simulink model "SD2231_Lab1m"  (R2018b)
settings: Solver=ode45  StartTime=0.0  StopTime=inf  RelTol=1e-3  EnableMultiTasking=on
values from neighbouring files (symbols this model uses):
  K_brake = K_brake(3)    [initial.m]    (also in initialm.m)
  K_em = K_em(3)    [initial.m]    (also in initialm.m)
  Kd_brake = 0    [initial.m]    (also in initialm.m)
  Kd_brake_r = 0.01    [initialm.m]
  Kd_em = 0.0    (= 0)    [initial.m]    (also in initialm.m)
  Ki_brake = 0    [initial.m]    (also in initialm.m = 22.5)
  Ki_brake_r = 13.5    [initialm.m]
  Ki_em = 1.2    [initial.m]    (also in initialm.m = 12.5)
  Kp_brake = 0    [initial.m]    (also in initialm.m = 5.5)
  Kp_brake_r = 4.25    [initialm.m]
  Kp_em = 6.5    [initial.m]    (also in initialm.m = 2.5)
undefined symbols (not defined in the file or in its folder): ABS_slip_refF, ABS_slip_refR, DiscIntNeverNeededParam, TCS_slip_ref, Veh
libraries: CarMaker4SL x37, simulink x9, autolibmappedmotor x2
(part 1 of 2)
settings Model: ExtModeAutoUpdateStatusClock=off  Creator=fh  LastModifiedBy=anirv
settings DataIOCC: LimitDataPoints=on  SaveFormat=Array  SignalLoggingName=sigsOut
settings OptimizationCC: BooleanDataType=off  ExpressionDepthLimit=2147483647  InitFltsAndDblsToZero=on  LifeSpan=inf
settings DebuggingCC: SaveWithParameterizedLinksMsg=none  UnderspecifiedInitializationDetection=Classic  MergeDetectMultiDrivingBlocksExec=none  SignalResolutionControl=TryResolveAllWithWarning  MultiTaskDSMMsg=warning  MultiTaskCondExecSysMsg=none  FcnCallInpInsideContextMsg=warning  StateNameClashWarn=warning  SFUnexpectedBacktrackingDiag=warning  SFNoUnconditionalDefaultTransitionDiag=warning
settings HardwareCC: ProdBitPerPointer=32  ProdBitPerSizeT=32  ProdBitPerPtrDiffT=32  ProdLargestAtomicFloat=None  ProdIntDivRoundTo=Undefined  ProdEndianess=Unspecified  ProdWordSize=32  ProdHWDeviceType=32-bit Generic  TargetUnknown=on
settings ModelReferenceCC: PropagateSignalLabelsOutOfModel=off
settings SFSimCC: SimUseLocalCustomCode=off
settings RTWCC: RTWUseLocalCustomCode=off
settings CodeAppCC: MaxIdLength=63  StateflowObjectComments=on
settings GRTTargetCC: TargetFcnLib=ansi_tfl_tmw.mat  TargetLangStandard=C89/C90 (ANSI)  GeneratePreprocessorConditionals=Disable all  CombineOutputUpdateFcns=off  GRTInterface=on
settings ConfigComp: CovMetricSettings=dw  CovHtmlReporting=on  CovSaveCumulativeToWorkspaceVar=on  CovSaveSingleToWorkspaceVar=on  CovExternalEMLEnable=off

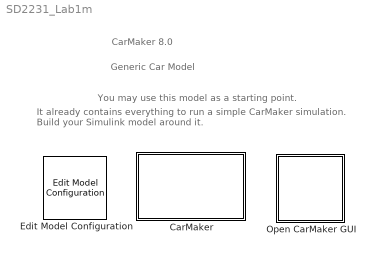
== system SD2231_Lab1m ==
  note: Generic Car Model
  note: You may use this model as a starting point.
  note: It already contains everything to run a simple CarMaker simulation.
      | Build your Simulink model around it.
  note: CarMaker 8.0
  CarMaker : Subsystem  TreatAsAtomicUnit=on
      mask Display: image(imread('CarMakerSys.png'));
  Edit Model Configuration : CarMaker4SL/Edit Model Configuration  SFunctionModules=''
  Open CarMaker GUI : Subsystem  LoadFcn=if ~length(which('cmself')), cmenv; end
      settings: OpenFcn=cmblockmagic('gui_fix_display'); CM_Simulink
      mask Display: image(imread('CarMakerGUI.png'));

== system SD2231_Lab1m/CarMaker ==
  Bus Creator : BusCreator  Inputs=6
  CM_FIRST : Subsystem
  CM_LAST : Subsystem
  CarMaker data : Subsystem
  DrivMan : Subsystem
  Ground : Ground
  IPG Vehicle : Subsystem  TreatAsAtomicUnit=on
  Road friction : Subsystem
  Terminator : Terminator
  Used friction mapping : Subsystem
  VehicleControl : Subsystem
  Your ABS Controller : Subsystem
  Your Traction Controller : Subsystem
  Your observer : Subsystem
  wires:
  DrivMan/2(DrivMan.Out) -> VehicleControl/2(DrivMan.In)
  DrivMan/1(Sync_Out) -> VehicleControl/1(Sync_In)
  CM_FIRST/2(Env.Misc) -> DrivMan/2(Env.Misc)
  CM_FIRST/1(Sync_Out) -> DrivMan/1(Sync_In)
  CM_LAST/1(Sync_Out) -> Terminator/1
  Ground/1 -> CM_FIRST/1(Sync_In)
  IPG Vehicle/1(Sync_Out) -> CM_LAST/1(Sync_In)
  VehicleControl/1(Sync_Out) -> IPG Vehicle/1(Sync_In)
  VehicleControl/3(VhclCtrl.Steering) -> IPG Vehicle/3(VhclCtrl.Steering)
  VehicleControl/4(Vhcl.Wheel.In) -> IPG Vehicle/4(Vhcl.Wheel.In)
  VehicleControl/5(Vhcl.Misc) -> IPG Vehicle/5(Vhcl.Misc)
  VehicleControl/6(VhclCtrl.Brake) -> IPG Vehicle/6(VhclCtrl.Brake)
  VehicleControl/7(VhclCtrl.PT) -> IPG Vehicle/7(VhclCtrl.PT)
  VehicleControl/2(Vhcl.Model.Source) -> IPG Vehicle/2(Vhcl.Model.Source)
  Your ABS Controller/1(FLBrakeAdjust (0-1)) -> Bus Creator/3
  Your ABS Controller/2(FRBrakeAdjust (0-1)) -> Bus Creator/4
  Your ABS Controller/3(RLBrakeAdjust (0-1)) -> Bus Creator/5
  Your ABS Controller/4(RRBrakeAdjust (0-1)) -> Bus Creator/6
  Bus Creator/1 -> IPG Vehicle/8(SD2231.data)
  CarMaker data/1(CarMaker bus data) -> Your observer/1(CarMaker bus data)
  Your observer/1(CarMaker bus data out) -> Your ABS Controller/1(CarMaker Bus data), Your Traction Controller/1(CarMaker Bus data)
  Your observer/2(Tyre slip bus data out) -> Your ABS Controller/2(TyreSlipBusDataOut), Your Traction Controller/2("TyreSlipBusDataOut "), Used friction mapping/1(Tyre slip bus data out)
  Your Traction Controller/1(LR TrqReqSignal (0-1)) -> Bus Creator/1
  Your Traction Controller/2(RR TrqReqSignal (0-1)) -> Bus Creator/2

== system SD2231_Lab1m/Open CarMaker GUI ==
  S-Function : S-Function  FunctionName=cm_gui  SFunctionDeploymentMode=off  EnableBusSupport=off

== system SD2231_Lab1m/CarMaker/CM_FIRST ==
  Sync_In : Inport
  BusCreator1 : BusCreator  Inputs=8
  BusCreator2 : BusCreator  Inputs=6
  Demux1 : Demux  Outputs=14
  Environment : S-Function  FunctionName=CM_Sfun  Parameters='Environment'  SFunctionDeploymentMode=off  EnableBusSupport=off
  IoIn : S-Function  FunctionName=CM_Sfun  Parameters='IoIn'  SFunctionDeploymentMode=off  EnableBusSupport=off
  Terminator : Terminator
  Sync_Out : Outport
  Env.Misc : Outport  Port=2
  wires:
  BusCreator2/1 -> Terminator/1  "IF Environment (in)"
  BusCreator1/1 -> Env.Misc/1
  Demux1/14 -> BusCreator2/6  "Env sRoad"
  Demux1/13 -> BusCreator2/5  "Env PoI_GCS Elev"
  Demux1/12 -> BusCreator2/4  "Env PoI_GCS Lat"
  Demux1/11 -> BusCreator2/3  "Env PoI_GCS Long"
  Demux1/10 -> BusCreator2/2  "Env Time"
  Demux1/9 -> BusCreator2/1  "Env yDay"
  Demux1/8 -> BusCreator1/8  "Env WindVel_tot z"
  Demux1/7 -> BusCreator1/7  "Env WindVel_tot y"
  Demux1/6 -> BusCreator1/6  "Env WindVel_tot x"
  Demux1/5 -> BusCreator1/5  "Env SolarRadiation"
  Demux1/4 -> BusCreator1/4  "Env AirHumidity"
  Demux1/3 -> BusCreator1/3  "Env AirPressure"
  Demux1/2 -> BusCreator1/2  "Env AirDensity"
  Demux1/1 -> BusCreator1/1  "Env Temperature"
  Environment/2 -> Demux1/1
  Environment/1 -> Sync_Out/1
  IoIn/1 -> Environment/1
  Sync_In/1 -> IoIn/1

== system SD2231_Lab1m/CarMaker/CM_LAST ==
  Sync_In : Inport
  CM_User : S-Function  FunctionName=CM_Sfun  Parameters='CM_User'  SFunctionDeploymentMode=off  EnableBusSupport=off
  IoOut : S-Function  FunctionName=CM_Sfun  Parameters='IoOut'  SFunctionDeploymentMode=off  EnableBusSupport=off
  Sync_Out : Outport
  wires:
  IoOut/1 -> Sync_Out/1
  CM_User/1 -> IoOut/1
  Sync_In/1 -> CM_User/1

== system SD2231_Lab1m/CarMaker/CarMaker data ==
  Brake pedal [0-1] : CarMaker4SL/Read CM Dict  xname=Driver.Brake  xsync=off
  Bus Creator : BusCreator  Inputs=15
  Distance [m] : CarMaker4SL/Read CM Dict  xname=Vhcl.Distance  xsync=off
  FL Tyre radius [m] : CarMaker4SL/Read CM Dict  xname=Car.WFL.Radius  xsync=off
  FL Tyre rot. vel. [rad/s] : CarMaker4SL/Read CM Dict  xname=Car.WheelSpd_FL  xsync=off
  FR Tyre radius [m] : CarMaker4SL/Read CM Dict  xname=Car.WFR.Radius  xsync=off
  FR Tyre rot. vel. [rad/s] : CarMaker4SL/Read CM Dict  xname=Car.WheelSpd_FR  xsync=off
  RL Tyre radius [m] : CarMaker4SL/Read CM Dict  xname=Car.WRL.Radius  xsync=off
  RL Tyre rot. vel. [rad/s] : CarMaker4SL/Read CM Dict  xname=Car.WheelSpd_RL  xsync=off
  RR Tyre radius [m] : CarMaker4SL/Read CM Dict  xname=Car.WRR.Radius  xsync=off
  RR Tyre rot. vel. [rad/s] : CarMaker4SL/Read CM Dict  xname=Car.WheelSpd_RR  xsync=off
  Steering wheel angle [rad] : CarMaker4SL/Read CM Dict  xname=Driver.Steer.Ang  xsync=off
  Throttle [0-1] : CarMaker4SL/Read CM Dict  xname=Driver.Gas  xsync=off
  Vehicle Yaw Rate [rad/s] : CarMaker4SL/Read CM Dict  xname=Car.YawRate  xsync=off
  Vehicle ax [m/s^2] : CarMaker4SL/Read CM Dict  xname=Car.ax  xsync=off
  Vehicle velocity [m/s] : CarMaker4SL/Read CM Dict  xname=Car.v  xsync=off
  CarMaker bus data : Outport
  wires:
  RR Tyre rot. vel. [rad/s]/1 -> Bus Creator/8  "RR Tyre rot vel"
  RL Tyre rot. vel. [rad/s]/1 -> Bus Creator/7  "RL Tyre rot vel"
  Distance [m]/1 -> Bus Creator/4  "Distance"
  FR Tyre rot. vel. [rad/s]/1 -> Bus Creator/6  "FR Tyre rot vel"
  Brake pedal [0-1]/1 -> Bus Creator/2  "Brake pedal"
  Vehicle ax [m/s^2]/1 -> Bus Creator/9  "Vehicle ax"
  Steering wheel angle [rad]/1 -> Bus Creator/3  "Steering wheel angle"
  Throttle [0-1]/1 -> Bus Creator/1  "Throttle"
  Vehicle velocity [m/s]/1 -> Bus Creator/10  "Vehicle velocity"
  FL Tyre rot. vel. [rad/s]/1 -> Bus Creator/5  "FL Tyre rot vel"
  Vehicle Yaw Rate [rad/s]/1 -> Bus Creator/11  "Vehicle Yaw Rate"
  FL Tyre radius [m]/1 -> Bus Creator/12  "FL Tyre radius"
  FR Tyre radius [m]/1 -> Bus Creator/13  "FR Tyre radius"
  RL Tyre radius [m]/1 -> Bus Creator/14  "RL Tyre radius"
  RR Tyre radius [m]/1 -> Bus Creator/15  "RR Tyre radius"
  Bus Creator/1 -> CarMaker bus data/1  "CarMaker bus data"

== system SD2231_Lab1m/CarMaker/DrivMan ==
  note: There's rarely a reason to override DrivMan signals.
      | Use the VehicleControl interface for this purpose.
  Sync_In : Inport
  Env.Misc : Inport  Port=2
  BusCreator : BusCreator  Inputs=17
  Demux : Demux  Outputs=17
  DrivMan : S-Function  FunctionName=CM_Sfun  Parameters='DrivMan'  SFunctionDeploymentMode=off  EnableBusSupport=off
  Sync_Out : Outport
  DrivMan.Out : Outport  Port=2
  wires:
  Demux/17 -> BusCreator/17  "DrivMan Steering Trq"
  Demux/16 -> BusCreator/16  "DrivMan Steering AngAcc"
  Demux/15 -> BusCreator/15  "DrivMan Steering AngVel"
  Demux/14 -> BusCreator/14  "DrivMan Steering Ang"
  Demux/13 -> BusCreator/13  "DrivMan Gas"
  Demux/12 -> BusCreator/12  "DrivMan Clutch"
  Demux/11 -> BusCreator/11  "DrivMan BrakePark"
  Demux/10 -> BusCreator/10  "DrivMan Brake"
  Demux/9 -> BusCreator/9  "DrivMan GearNo"
  Demux/8 -> BusCreator/8  "DrivMan SelectorCtrl"
  Demux/7 -> BusCreator/7  "DrivMan UserSignal4"
  Demux/6 -> BusCreator/6  "DrivMan UserSignal3"
  Demux/5 -> BusCreator/5  "DrivMan UserSignal2"
  Demux/4 -> BusCreator/4  "DrivMan UserSignal1"
  Demux/3 -> BusCreator/3  "DrivMan UserSignal0"
  Demux/2 -> BusCreator/2  "DrivMan Key"
  Demux/1 -> BusCreator/1  "DrivMan SST"
  Env.Misc/1 -> DrivMan/2
  Sync_In/1 -> DrivMan/1
  DrivMan/1 -> Sync_Out/1
  BusCreator/1 -> DrivMan.Out/1
  DrivMan/2 -> Demux/1

== system SD2231_Lab1m/CarMaker/IPG Vehicle ==
  Sync_In : Inport
  Vhcl.Model.Source : Inport  Port=2
  VhclCtrl.Steering : Inport  Port=3
  Vhcl.Wheel.In : Inport  Port=4
  Vhcl.Misc : Inport  Port=5
  VhclCtrl.Brake : Inport  Port=6
  VhclCtrl.PT : Inport  Port=7
  SD2231.data : Inport  Port=8
  Brake1 : Subsystem
  CarAndTrailer1 : Subsystem
  PowerTrain1 : Subsystem
  Stop Simulation : Stop
  VehicleSource_BuiltIn : simulink/Logic and Bit Operations/Compare To Constant  relop=~=  const=1  OutDataTypeStr=boolean  ZeroCross=off
  Sync_Out : Outport
  wires:
  CarAndTrailer1/1(Sync_Out) -> Brake1/1(Sync_In)
  CarAndTrailer1/2(Brake.IF.In) -> Brake1/2(Brake.IF.In)
  VhclCtrl.Brake/1 -> Brake1/3(VhclCtrl.Brake)
  PowerTrain1/1(Sync_Out) -> Sync_Out/1
  Vhcl.Misc/1 -> CarAndTrailer1/4(Vhcl.Misc)
  Vhcl.Wheel.In/1 -> CarAndTrailer1/3(Vhcl.Wheel.In)
  VhclCtrl.Steering/1 -> CarAndTrailer1/2(VhclCtrl.Steering)
  Sync_In/1 -> CarAndTrailer1/1(Sync_In)
  Vhcl.Model.Source/1 -> VehicleSource_BuiltIn/1
  VehicleSource_BuiltIn/1 -> Stop Simulation/1
  Brake1/1(Sync_Out) -> PowerTrain1/1(Sync_In)
  Brake1/2(Vhcl.Wheel.PT) -> PowerTrain1/2(Vhcl.Wheel.PT)
  VhclCtrl.PT/1 -> PowerTrain1/3(VhclCtrl.PT)
  Brake1/3(Brake.IF.Out) -> PowerTrain1/4(Brake.IF.Out)
  CarAndTrailer1/3(Car.Trq_T2W) -> PowerTrain1/5(Car.TrqT2W)
  SD2231.data/1 -> Brake1/4(SD2231.Data), PowerTrain1/6(SD2232.data)

== system SD2231_Lab1m/CarMaker/Road friction ==
  Constant : Constant  Value=Veh.mu
  Write CM Dict : CarMaker4SL/Write CM Dict  xname=Car.muRoadFL  xsync=off
  Write CM Dict1 : CarMaker4SL/Write CM Dict  xname=Car.muRoadFR  xsync=off
  Write CM Dict2 : CarMaker4SL/Write CM Dict  xname=Car.muRoadRL  xsync=off
  Write CM Dict3 : CarMaker4SL/Write CM Dict  xname=Car.muRoadRR  xsync=off
  wires:
  Constant/1 -> Write CM Dict3/1, Write CM Dict2/1, Write CM Dict1/1, Write CM Dict/1

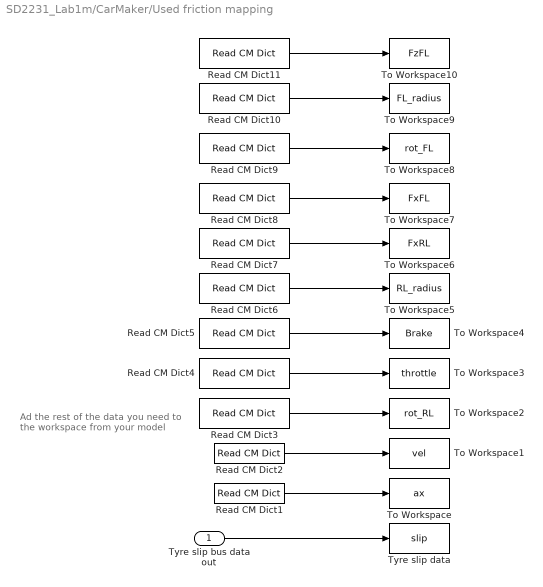
== system SD2231_Lab1m/CarMaker/Used friction mapping ==
  note: Ad the rest of the data you need to
      | the workspace from your model
  Tyre slip bus data out : Inport
  Read CM Dict1 : CarMaker4SL/Read CM Dict  xname=Car.ax  xsync=off
  Read CM Dict10 : CarMaker4SL/Read CM Dict  xname=Car.WRL.Radius  xsync=off
  Read CM Dict11 : CarMaker4SL/Read CM Dict  xname=Car.FzFL  xsync=off
  Read CM Dict2 : CarMaker4SL/Read CM Dict  xname=Car.v  xsync=off
  Read CM Dict3 : CarMaker4SL/Read CM Dict  xname=Car.WheelSpd_RL  xsync=off
  Read CM Dict4 : CarMaker4SL/Read CM Dict  xname=Driver.Gas  xsync=off
  Read CM Dict5 : CarMaker4SL/Read CM Dict  xname=Driver.Brake  xsync=off
  Read CM Dict6 : CarMaker4SL/Read CM Dict  xname=Car.WRL.Radius  xsync=off
  Read CM Dict7 : CarMaker4SL/Read CM Dict  xname=Car.FxRL  xsync=off
  Read CM Dict8 : CarMaker4SL/Read CM Dict  xname=Car.FxFL  xsync=off
  Read CM Dict9 : CarMaker4SL/Read CM Dict  xname=Car.WheelSpd_FL  xsync=off
  To Workspace : ToWorkspace  VariableName=ax  SampleTime=-1
  To Workspace1 : ToWorkspace  VariableName=vel  SampleTime=-1
  To Workspace10 : ToWorkspace  VariableName=FzFL  SampleTime=-1
  To Workspace2 : ToWorkspace  VariableName=rot_RL  SampleTime=-1
  To Workspace3 : ToWorkspace  VariableName=throttle  SampleTime=-1
  To Workspace4 : ToWorkspace  VariableName=Brake  SampleTime=-1
  To Workspace5 : ToWorkspace  VariableName=RL_radius  SampleTime=-1
  To Workspace6 : ToWorkspace  VariableName=FxRL  SampleTime=-1
  To Workspace7 : ToWorkspace  VariableName=FxFL  SampleTime=-1
  To Workspace8 : ToWorkspace  VariableName=rot_FL  SampleTime=-1
  To Workspace9 : ToWorkspace  VariableName=FL_radius  SampleTime=-1
  Tyre slip data : ToWorkspace  VariableName=slip  SampleTime=-1
  wires:
  Read CM Dict1/1 -> To Workspace/1
  Tyre slip bus data out/1 -> Tyre slip data/1
  Read CM Dict2/1 -> To Workspace1/1
  Read CM Dict3/1 -> To Workspace2/1
  Read CM Dict4/1 -> To Workspace3/1
  Read CM Dict5/1 -> To Workspace4/1
  Read CM Dict6/1 -> To Workspace5/1
  Read CM Dict8/1 -> To Workspace7/1
  Read CM Dict7/1 -> To Workspace6/1
  Read CM Dict9/1 -> To Workspace8/1
  Read CM Dict10/1 -> To Workspace9/1
  Read CM Dict11/1 -> To Workspace10/1

== system SD2231_Lab1m/CarMaker/VehicleControl ==
  note: <Your model here>
  note: When implementing a vehicle control model,
      | be sure to add '-disablevehiclecontrol' to the command line arguments
      | in the CarMaker Model Configuration block.
      | Otherwise your model will possibly not see the original DrivMan signals
      | on its inputs, but those of a currently activated C-coded vehicle control model instead.
  Sync_In : Inport
  DrivMan.In : Inport  Port=2
  Bus Creator2 : BusCreator  Inputs=2
  CreateBus Vhcl.Misc : Subsystem
  CreateBus Vhcl.Wheel.In : Subsystem
  CreateBus VhclCtrl : Subsystem
  CreateBus VhclCtrl.PT : Subsystem
  CreateBus VhclCtrl.Steering : Subsystem
  Demux2 : Demux  Outputs=2
  VehicleControl : S-Function  FunctionName=CM_Sfun  Parameters='VehicleControl'  SFunctionDeploymentMode=off  EnableBusSupport=off
  VehicleControlUpd : S-Function  FunctionName=CM_Sfun  Parameters='VehicleControlUpd'  SFunctionDeploymentMode=off  EnableBusSupport=off
  Sync_Out : Outport
  Vhcl.Model.Source : Outport  Port=2
  VhclCtrl.Steering : Outport  Port=3
  Vhcl.Wheel.In : Outport  Port=4
  Vhcl.Misc : Outport  Port=5
  VhclCtrl.Brake : Outport  Port=6
  VhclCtrl.PT : Outport  Port=7
  wires:
  CreateBus VhclCtrl/1(Out) -> VehicleControlUpd/2
  VehicleControl/2 -> CreateBus VhclCtrl/1(In)
  VehicleControlUpd/2 -> Vhcl.Model.Source/1
  VehicleControlUpd/4 -> CreateBus Vhcl.Wheel.In/1(In1)
  VehicleControlUpd/5 -> CreateBus Vhcl.Misc/1(In1)
  VehicleControlUpd/6 -> Demux2/1
  VehicleControlUpd/7 -> CreateBus VhclCtrl.PT/1(In1)
  VehicleControlUpd/3 -> CreateBus VhclCtrl.Steering/1(In1)
  CreateBus Vhcl.Misc/1(Out1) -> Vhcl.Misc/1
  CreateBus Vhcl.Wheel.In/1(Out1) -> Vhcl.Wheel.In/1
  DrivMan.In/1 -> VehicleControl/2
  VehicleControl/1 -> VehicleControlUpd/1
  Sync_In/1 -> VehicleControl/1
  CreateBus VhclCtrl.PT/1(Out1) -> VhclCtrl.PT/1
  Bus Creator2/1 -> VhclCtrl.Brake/1
  CreateBus VhclCtrl.Steering/1(Out1) -> VhclCtrl.Steering/1
  VehicleControlUpd/1 -> Sync_Out/1
  Demux2/2 -> Bus Creator2/2  "VhclCtrl BrakePark"
  Demux2/1 -> Bus Creator2/1  "VhclCtrl Brake"

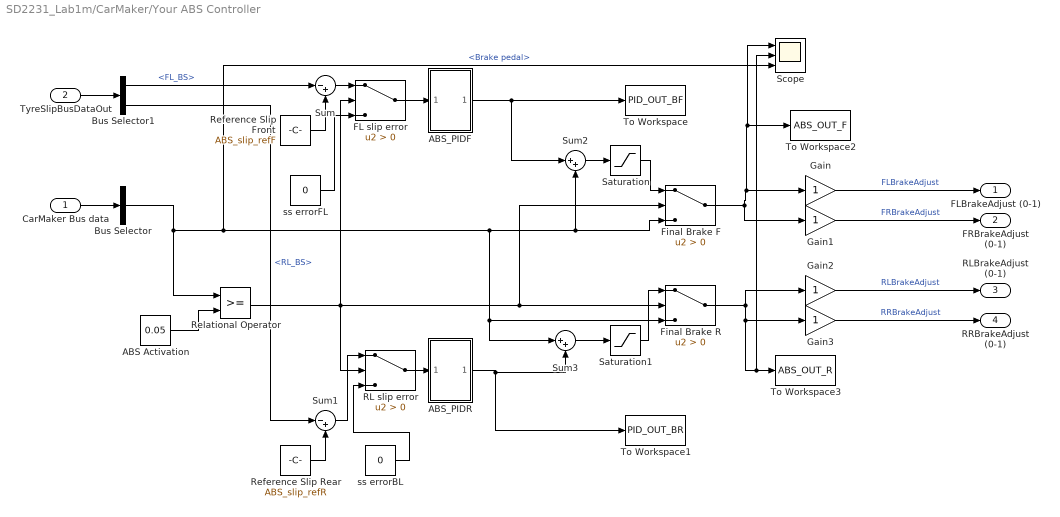
== system SD2231_Lab1m/CarMaker/Your ABS Controller ==
  CarMaker Bus data : Inport
  TyreSlipBusDataOut : Inport  Port=2
  ABS Activation : Constant  Value=0.05
  ABS_PIDF : Subsystem
  ABS_PIDR : Subsystem
  Bus Selector : BusSelector  OutputSignals=Brake pedal
  Bus Selector1 : BusSelector  OutputSignals=FL_BS,RL_BS
  FL slip error : Switch  Criteria=u2 > Threshold
  Final Brake F : Switch  Criteria=u2 > Threshold
  Final Brake R : Switch  Criteria=u2 > Threshold
  Gain{,1..3} (4 alike) : Gain
  RL slip error : Switch  Criteria=u2 > Threshold
  Reference Slip Rear : Constant  Value=ABS_slip_refR
  Reference Slip Front : Constant  Value=ABS_slip_refF
  Relational Operator : RelationalOperator  OutDataTypeStr=boolean  RndMeth=Simplest
  Saturation : Saturate  UpperLimit=1  LowerLimit=0  LinearizeAsGain=off  ZeroCross=off
  Saturation1 : Saturate  UpperLimit=1  LowerLimit=0  LinearizeAsGain=off  ZeroCross=off
  Scope : Scope  NumInputPorts=3
  Sum : Sum  Inputs=|-+
  Sum1 : Sum  Inputs=|-+
  Sum2 : Sum  Inputs=|++
  Sum3 : Sum  Inputs=|++
  To Workspace : ToWorkspace  VariableName=PID_OUT_BF  SaveFormat=Timeseries  SampleTime=-1
  To Workspace1 : ToWorkspace  VariableName=PID_OUT_BR  SaveFormat=Timeseries  SampleTime=-1
  To Workspace2 : ToWorkspace  VariableName=ABS_OUT_F  SaveFormat=Timeseries  SampleTime=-1
  To Workspace3 : ToWorkspace  VariableName=ABS_OUT_R  SaveFormat=Timeseries  SampleTime=-1
  ss errorBL : Constant  Value=0
  ss errorFL : Constant  Value=0
  FLBrakeAdjust (0-1) : Outport
  FRBrakeAdjust (0-1) : Outport  Port=2
  RLBrakeAdjust (0-1) : Outport  Port=3
  RRBrakeAdjust (0-1) : Outport  Port=4
  wires:
  CarMaker Bus data/1 -> Bus Selector/1
  Gain/1 -> FLBrakeAdjust (0-1)/1  "FLBrakeAdjust"
  Gain1/1 -> FRBrakeAdjust (0-1)/1  "FRBrakeAdjust"
  Gain2/1 -> RLBrakeAdjust (0-1)/1  "RLBrakeAdjust"
  Gain3/1 -> RRBrakeAdjust (0-1)/1  "RRBrakeAdjust"
  ABS Activation/1 -> Relational Operator/2
  TyreSlipBusDataOut/1 -> Bus Selector1/1
  Reference Slip Front/1 -> Sum/2
  Reference Slip Rear/1 -> Sum1/2
  Relational Operator/1 -> RL slip error/2, Final Brake R/2, Final Brake F/2, FL slip error/2
  ABS_PIDR/1(Out1) -> Sum3/2, To Workspace1/1
  Bus Selector1/1 -> Sum/1  "<FL_BS>"
  Bus Selector/1 -> Relational Operator/1, Scope/3, Sum3/1, Final Brake R/3, Sum2/2, Final Brake F/3  "<Brake pedal>"
  Bus Selector1/2 -> Sum1/1  "<RL_BS>"
  Final Brake F/1 -> Scope/1, To Workspace2/1, Gain/1, Gain1/1
  Final Brake R/1 -> Scope/2, To Workspace3/1, Gain3/1, Gain2/1
  Sum2/1 -> Saturation/1
  Saturation/1 -> Final Brake F/1
  Sum3/1 -> Saturation1/1
  Saturation1/1 -> Final Brake R/1
  ss errorFL/1 -> FL slip error/3
  Sum/1 -> FL slip error/1
  FL slip error/1 -> ABS_PIDF/1(In1)
  Sum1/1 -> RL slip error/1
  RL slip error/1 -> ABS_PIDR/1(In1)
  ss errorBL/1 -> RL slip error/3
  ABS_PIDF/1(Out1) -> Sum2/1, To Workspace/1

== system SD2231_Lab1m/CarMaker/Your Traction Controller ==
  CarMaker Bus data : Inport
  "TyreSlipBusDataOut " : Inport  Port=2
  Bus Selector : BusSelector  OutputSignals=Throttle
  Bus Selector1 : BusSelector  OutputSignals=RL_TS
  Constant : Constant  Value=0
  Gain : Gain
  Gain1 : Gain
  Relational Operator : RelationalOperator  Operator=<=  OutDataTypeStr=boolean  RndMeth=Simplest
  SS error : Constant  Value=0
  Saturation : Saturate  UpperLimit=1  LowerLimit=0  LinearizeAsGain=off  ZeroCross=off
  "Slip Check " : Switch  Criteria=u2 > Threshold  Threshold=0.01
  Slip reference : Constant  Value=TCS_slip_ref
  Sum : Sum  Inputs=|-+
  Sum1 : Sum  Inputs=|++
  TCS Active : Switch  Criteria=u2 > Threshold  Threshold=0.4
  TCS_PID : Subsystem
  Throttle Check : Switch  Criteria=u2 > Threshold
  To Workspace : ToWorkspace  VariableName=PID_out  SaveFormat=Timeseries  SampleTime=-1
  To Workspace1 : ToWorkspace  VariableName=TCS_out  SaveFormat=Timeseries  SampleTime=-1
  LR TrqReqSignal (0-1) : Outport
  RR TrqReqSignal (0-1) : Outport  Port=2
  wires:
  CarMaker Bus data/1 -> Bus Selector/1
  Gain1/1 -> RR TrqReqSignal (0-1)/1  "RRTrqAdjust"
  Gain/1 -> LR TrqReqSignal (0-1)/1  "LRTrqAdjust"
  "TyreSlipBusDataOut "/1 -> Bus Selector1/1
  Bus Selector1/1 -> "Slip Check "/1, "Slip Check "/2  "<RL_TS>"
  Constant/1 -> "Slip Check "/3
  Slip reference/1 -> Sum/2
  "Slip Check "/1 -> Sum/1
  Sum/1 -> TCS Active/1
  Bus Selector/1 -> Throttle Check/3, Relational Operator/2, Sum1/2, TCS Active/2  "<Throttle>"
  SS error/1 -> TCS Active/3
  Throttle Check/1 -> Gain1/1, Gain/1, To Workspace1/1
  Sum1/1 -> Saturation/1
  Saturation/1 -> Throttle Check/1, Relational Operator/1
  Relational Operator/1 -> Throttle Check/2
  TCS_PID/1(Out1) -> To Workspace/1, Sum1/1
  TCS Active/1 -> TCS_PID/1(In1)

== system SD2231_Lab1m/CarMaker/Your observer ==
  note: Ad your own slip observer
  CarMaker bus data : Inport
  Bus Selector : BusSelector  OutputSignals=Vehicle velocity,RL Tyre rot vel,RL Tyre radius,FL Tyre rot vel,FL Tyre radius,RR Tyre rot vel,RR Tyre radius,FR Tyre rot vel,FR Tyre radius
  BusCreator : BusCreator  Inputs=8
  FL_observer : Subsystem
  FR_observer : Subsystem
  RL_observer : Subsystem
  RR_observer : Subsystem
  CarMaker bus data out : Outport
  Tyre slip bus data out : Outport  Port=2
  wires:
  CarMaker bus data/1 -> Bus Selector/1, CarMaker bus data out/1
  BusCreator/1 -> Tyre slip bus data out/1
  Bus Selector/1 -> FR_observer/1(<Vehicle velocity>), RR_observer/1(<Vehicle velocity>), FL_observer/1(<Vehicle velocity>), RL_observer/1(<Vehicle velocity>)  "<Vehicle velocity>"
  Bus Selector/4 -> FL_observer/2(<FL Tyre rot vel>)  "<FL Tyre rot vel>"
  Bus Selector/5 -> FL_observer/3(<FL Tyre radius>)  "<FL Tyre radius>"
  Bus Selector/6 -> RR_observer/2(<RR Tyre rot vel>)  "<RR Tyre rot vel>"
  Bus Selector/7 -> RR_observer/3(<RR Tyre radius>)  "<RR Tyre radius>"
  Bus Selector/8 -> FR_observer/2(<FR_RL Tyre rot vel>)  "<FR Tyre rot vel>"
  Bus Selector/9 -> FR_observer/3(<FR_RL Tyre radius>)  "<FR Tyre radius>"
  FL_observer/1(FL_BS) -> BusCreator/3  "FL_BS"
  FL_observer/2(FL_TS) -> BusCreator/4  "FL_TS"
  RR_observer/1(RR_BS) -> BusCreator/5  "RR_BS"
  RR_observer/2(RR_TS) -> BusCreator/6  "RR_TS"
  FR_observer/1(FR_BS) -> BusCreator/7  "FR_BS"
  FR_observer/2(FR_TS) -> BusCreator/8  "FR_TS"
  Bus Selector/2 -> RL_observer/2(<RL Tyre rot vel>)  "<RL Tyre rot vel>"
  Bus Selector/3 -> RL_observer/3(<RL Tyre radius>)  "<RL Tyre radius>"
  RL_observer/1(RL_BS) -> BusCreator/1  "RL_BS"
  RL_observer/2(RL_TS) -> BusCreator/2  "RL_TS"

== system SD2231_Lab1m/CarMaker/IPG Vehicle/Brake1 ==
  note: When replacing the entire braking system,
      | be sure to add '-disablebrake' to the command line arguments
      | in the CarMaker Model Configuration block.
  note: <Your model here>
  Sync_In : Inport
  Brake.IF.In : Inport  Port=2
  VhclCtrl.Brake : Inport  Port=3
  SD2231.Data : Inport  Port=4
  Brake : S-Function  FunctionName=CM_Sfun  Parameters='Brake'  SFunctionDeploymentMode=off  EnableBusSupport=off
  BrakeUpd : S-Function  FunctionName=CM_Sfun  Parameters='BrakeUpd'  SFunctionDeploymentMode=off  EnableBusSupport=off
  BusCreator1 : BusCreator  Inputs=16
  CreateBus Vhcl.Wheel.PT : Subsystem
  Demux : Demux  Outputs=16
  Terminator : Terminator
  UserDefinedBrakingSystem : Subsystem  TreatAsAtomicUnit=on
  Sync_Out : Outport
  Vhcl.Wheel.PT : Outport  Port=2
  Brake.IF.Out : Outport  Port=3
  wires:
  Demux/16 -> BusCreator1/16  "Brake IF Trq_DriveSrc_trg d3"
  Demux/15 -> BusCreator1/15  "Brake IF Trq_DriveSrc_trg d2"
  Demux/14 -> BusCreator1/14  "Brake IF Trq_DriveSrc_trg d1"
  Demux/13 -> BusCreator1/13  "Brake IF Trq_DriveSrc_trg d0"
  Demux/12 -> BusCreator1/12  "Brake IF Trq_Reg_trg RR"
  Demux/11 -> BusCreator1/11  "Brake IF Trq_Reg_trg RL"
  Demux/10 -> BusCreator1/10  "Brake IF Trq_Reg_trg FR"
  Demux/9 -> BusCreator1/9  "Brake IF Trq_Reg_trg FL"
  Demux/8 -> BusCreator1/8  "Brake IF Trq_PB RR"
  Demux/7 -> BusCreator1/7  "Brake IF Trq_PB RL"
  Demux/6 -> BusCreator1/6  "Brake IF Trq_PB FR"
  Demux/5 -> BusCreator1/5  "Brake IF Trq_PB FL"
  Demux/4 -> BusCreator1/4  "Brake IF Trq_WB RR"
  Demux/3 -> BusCreator1/3  "Brake IF Trq_WB RL"
  Demux/2 -> BusCreator1/2  "Brake IF Trq_WB FR"
  Demux/1 -> BusCreator1/1  "Brake IF Trq_WB FL"
  Brake/2 -> Terminator/1
  BusCreator1/1 -> BrakeUpd/2, Brake.IF.Out/1
  BrakeUpd/1 -> Sync_Out/1
  Brake/1 -> BrakeUpd/1  "Sync"
  Brake.IF.In/1 -> Brake/2
  VhclCtrl.Brake/1 -> Brake/3
  Sync_In/1 -> Brake/1
  BrakeUpd/2 -> CreateBus Vhcl.Wheel.PT/1(In)
  CreateBus Vhcl.Wheel.PT/1(Out) -> Vhcl.Wheel.PT/1
  SD2231.Data/1 -> UserDefinedBrakingSystem/1(SD2231.Data)
  UserDefinedBrakingSystem/1(Brake.IF.Out) -> Demux/1

== system SD2231_Lab1m/CarMaker/IPG Vehicle/CarAndTrailer1 ==
  Sync_In : Inport
  VhclCtrl.Steering : Inport  Port=2
  Vhcl.Wheel.In : Inport  Port=3
  Vhcl.Misc : Inport  Port=4
  CarAndTrailerUpd : Subsystem
  Forces : Subsystem
  Ground : Ground
  Kinematics : Subsystem
  Kinetics : Subsystem
  Steering : Subsystem
  Terminator : Terminator
  Terminator1 : Terminator
  Trailer : Subsystem
  Sync_Out : Outport
  Brake.IF.In : Outport  Port=2
  Car.Trq_T2W : Outport  Port=3
  wires:
  Trailer/9(Car.Hitch.FrcTrq) -> CarAndTrailerUpd/9(Car.Hitch.FrcTrq)
  Trailer/8(Vhcl.Wheel.RR) -> CarAndTrailerUpd/8(Vhcl.Wheel.RR)
  Trailer/7(Vhcl.Wheel.RL) -> CarAndTrailerUpd/7(Vhcl.Wheel.RL)
  Trailer/6(Vhcl.Wheel.FR) -> CarAndTrailerUpd/6(Vhcl.Wheel.FR)
  Trailer/5(Vhcl.Wheel.FL) -> CarAndTrailerUpd/5(Vhcl.Wheel.FL)
  Trailer/4(Vhcl.PoI) -> CarAndTrailerUpd/4(Vhcl.PoI)
  Trailer/3(Vhcl.Motion) -> CarAndTrailerUpd/3(Vhcl.Motion)
  Trailer/2(Vhcl.Steering) -> CarAndTrailerUpd/2(Vhcl.Steering)
  Trailer/1(Sync_Out) -> CarAndTrailerUpd/1(Sync_In)
  CarAndTrailerUpd/2(Brake.IF.In) -> Brake.IF.In/1
  CarAndTrailerUpd/1(Sync_Out) -> Sync_Out/1
  Vhcl.Misc/1 -> Terminator1/1
  Vhcl.Wheel.In/1 -> Terminator/1
  Kinetics/6(WheelCarrier.Misc) -> Trailer/6(WheelCarrier.Misc)
  Kinetics/5(Car.Trq_T2W) -> Trailer/5(Car.Trq_T2W), Car.Trq_T2W/1
  Steering/2(Steer.IF) -> Kinematics/2(Steer.IF)
  Kinetics/4(Car.Fr1) -> Trailer/4(Car.Fr1)
  Kinetics/3(Car.Hitch) -> Trailer/3(Car.Hitch)
  Kinetics/2(Trailer.Load) -> Trailer/2(Trailer.Load)
  VhclCtrl.Steering/1 -> Steering/2(VhclCtrl.Steering)
  Sync_In/1 -> Steering/1(Sync_In)
  Steering/1(Sync_Out) -> Kinematics/1(Sync_In)
  Kinetics/1(Sync_Out) -> Trailer/1(Sync_In)
  Ground/1 -> CarAndTrailerUpd/10(Vhcl.Fr1A)
  Forces/11(FStabi) -> Kinetics/11(FStabi)
  Forces/10(FDamp) -> Kinetics/10(FDamp)
  Forces/9(FSpring) -> Kinetics/9(FSpring)
  Forces/8(TireRR_Out) -> Kinetics/8(TireRR.Out)
  Forces/7(TireRL_Out) -> Kinetics/7(TireRL.Out)
  Forces/6(TireFR_Out) -> Kinetics/6(TireFR.Out)
  Forces/5(TireFL_Out) -> Kinetics/5(TireFL.Out)
  Forces/4(Car.Load) -> Kinetics/4(Car.Load)
  Forces/2(Car.Virtual) -> Kinetics/2(Car.Virtual)
  Kinematics/6(lSpring) -> Forces/6(lSpring)
  Kinematics/7(vDamp) -> Forces/7(vDamp)
  Forces/3(Car.Aero) -> Kinetics/3(Car.Aero)
  Forces/1(Sync_Out) -> Kinetics/1(Sync_In)
  Kinematics/5(TireRR_In) -> Forces/5(TireRR_In)
  Kinematics/4(TireRL_In) -> Forces/4(TireRL_In)
  Kinematics/3(TireFR_In) -> Forces/3(TireFR_In)
  Kinematics/2(TireFL_In) -> Forces/2(TireFL_In)
  Kinematics/1(Sync_Out) -> Forces/1(Sync_In)
  Kinematics/8(lStabi) -> Forces/8(lStabi)
  Forces/12(FBuf) -> Kinetics/12(FBuf)
  Kinematics/9(lBuf) -> Forces/9(lBuf)

== system SD2231_Lab1m/CarMaker/IPG Vehicle/PowerTrain1 ==
  note: When replacing the entire powertrain,
      | be sure to add '-disablepowertrain' to the command line arguments
      | in the CarMaker Model Configuration block.
  Sync_In : Inport
  Vhcl.Wheel.PT : Inport  Port=2
  VhclCtrl.PT : Inport  Port=3
  Brake.IF.Out : Inport  Port=4
  Car.TrqT2W : Inport  Port=5
  SD2232.data : Inport  Port=6
  BusCreator1 : BusCreator  Inputs=42
  Demux1 : Demux  Outputs=42
  PowerTrain : S-Function  FunctionName=CM_Sfun  Parameters='PowerTrain'  SFunctionDeploymentMode=off  EnableBusSupport=off
  PowerTrainUpd : S-Function  FunctionName=CM_Sfun  Parameters='PowerTrainUpd'  SFunctionDeploymentMode=off  EnableBusSupport=off
  Terminator : Terminator
  User RearDriven PowerTrain1 : Subsystem
  Sync_Out : Outport
  wires:
  Demux1/42 -> BusCreator1/42  "PT IF WRR Trq_BrakeReg_max"
  Demux1/41 -> BusCreator1/41  "PT IF WRR Trq_BrakeReg"
  Demux1/40 -> BusCreator1/40  "PT IF WRR Trq_Supp2WC"
  Demux1/39 -> BusCreator1/39  "PT IF WRR Trq_Drive"
  Demux1/38 -> BusCreator1/38  "PT IF WRR Trq_B2W"
  Demux1/37 -> BusCreator1/37  "PT IF WRR rotv"
  Demux1/36 -> BusCreator1/36  "PT IF WRR rot"
  Demux1/35 -> BusCreator1/35  "PT IF WRL Trq_BrakeReg_max"
  Demux1/34 -> BusCreator1/34  "PT IF WRL Trq_BrakeReg"
  Demux1/33 -> BusCreator1/33  "PT IF WRL Trq_Supp2WC"
  Demux1/32 -> BusCreator1/32  "PT IF WRL Trq_Drive"
  Demux1/31 -> BusCreator1/31  "PT IF WRL Trq_B2W"
  Demux1/30 -> BusCreator1/30  "PT IF WRL rotv"
  Demux1/29 -> BusCreator1/29  "PT IF WRL rot"
  Demux1/28 -> BusCreator1/28  "PT IF WFR Trq_BrakeReg_max"
  Demux1/27 -> BusCreator1/27  "PT IF WFR Trq_BrakeReg"
  Demux1/26 -> BusCreator1/26  "PT IF WFR Trq_Supp2WC"
  Demux1/25 -> BusCreator1/25  "PT IF WFR Trq_Drive"
  Demux1/24 -> BusCreator1/24  "PT IF WFR Trq_B2W"
  Demux1/23 -> BusCreator1/23  "PT IF WFR rotv"
  Demux1/22 -> BusCreator1/22  "PT IF WFR rot"
  Demux1/21 -> BusCreator1/21  "PT IF WFL Trq_BrakeReg_max"
  Demux1/20 -> BusCreator1/20  "PT IF WFL Trq_BrakeReg"
  Demux1/19 -> BusCreator1/19  "PT IF WFL Trq_Supp2WC"
  Demux1/18 -> BusCreator1/18  "PT IF WFL Trq_Drive"
  Demux1/17 -> BusCreator1/17  "PT IF WFL Trq_B2W"
  Demux1/16 -> BusCreator1/16  "PT IF WFL rotv"
  Demux1/15 -> BusCreator1/15  "PT IF WFL rot"
  Demux1/14 -> BusCreator1/14  "PT IF DL_iDiff_mean"
  Demux1/13 -> BusCreator1/13  "PT IF Trq_Supp2BdyEng y"
  Demux1/12 -> BusCreator1/12  "PT IF Trq_Supp2BdyEng x"
  Demux1/11 -> BusCreator1/11  "PT IF Trq_Supp2Bdy1B z"
  Demux1/10 -> BusCreator1/10  "PT IF Trq_Supp2Bdy1B y"
  Demux1/9 -> BusCreator1/9  "PT IF Trq_Supp2Bdy1B x"
  Demux1/8 -> BusCreator1/8  "PT IF Trq_Supp2Bdy1 z"
  Demux1/7 -> BusCreator1/7  "PT IF Trq_Supp2Bdy1 y"
  Demux1/6 -> BusCreator1/6  "PT IF Trq_Supp2Bdy1 x"
  Demux1/5 -> BusCreator1/5  "PT IF Engine_rotv"
  Demux1/4 -> BusCreator1/4  "PT IF GearNo"
  Demux1/3 -> BusCreator1/3  "PT IF OperationError"
  Demux1/2 -> BusCreator1/2  "PT IF OperationState"
  Demux1/1 -> BusCreator1/1  "PT IF Ignition"
  Sync_In/1 -> PowerTrain/1
  PowerTrain/2 -> Demux1/1
  PowerTrainUpd/1 -> Sync_Out/1
  PowerTrain/1 -> PowerTrainUpd/1  "Sync"
  VhclCtrl.PT/1 -> User RearDriven PowerTrain1/1(VhclCtrl), PowerTrain/3
  Vhcl.Wheel.PT/1 -> PowerTrain/2
  Car.TrqT2W/1 -> User RearDriven PowerTrain1/3(ResistanceTorques)
  Brake.IF.Out/1 -> User RearDriven PowerTrain1/2(BrakingTorques)
  SD2232.data/1 -> User RearDriven PowerTrain1/4(SD2231.data)
  BusCreator1/1 -> Terminator/1
  User RearDriven PowerTrain1/1(PowerTrainOut) -> PowerTrainUpd/2

== system SD2231_Lab1m/CarMaker/VehicleControl/CreateBus Vhcl.Misc ==
  In1 : Inport
  BusCreator : BusCreator  Inputs=11
  Demux : Demux  Outputs=11
  Out1 : Outport
  wires:
  Demux/11 -> BusCreator/11  "Vhcl Wind_vel_0 z"
  Demux/10 -> BusCreator/10  "Vhcl Wind_vel_0 y"
  Demux/9 -> BusCreator/9  "Vhcl Wind_vel_0 x"
  Demux/8 -> BusCreator/8  "Vhcl Trq_DL2BdyEng y"
  Demux/7 -> BusCreator/7  "Vhcl Trq_DL2BdyEng x"
  Demux/6 -> BusCreator/6  "Vhcl Trq_DL2Bdy1B z"
  Demux/5 -> BusCreator/5  "Vhcl Trq_DL2Bdy1B y"
  Demux/4 -> BusCreator/4  "Vhcl Trq_DL2Bdy1B x"
  Demux/3 -> BusCreator/3  "Vhcl Trq_DL2Bdy1 z"
  Demux/2 -> BusCreator/2  "Vhcl Trq_DL2Bdy1 y"
  Demux/1 -> BusCreator/1  "Vhcl Trq_DL2Bdy1 x"
  In1/1 -> Demux/1
  BusCreator/1 -> Out1/1

== system SD2231_Lab1m/CarMaker/VehicleControl/CreateBus Vhcl.Wheel.In ==
  In1 : Inport
  Bus Creator1 : BusCreator  Inputs=12
  Demux1 : Demux  Outputs=12
  Out1 : Outport
  wires:
  Demux1/12 -> Bus Creator1/12  "Vhcl Wheel RR rotv"
  Demux1/11 -> Bus Creator1/11  "Vhcl Wheel RR Trq_DL2WC"
  Demux1/10 -> Bus Creator1/10  "Vhcl Wheel RR Trq_B2WC"
  Demux1/9 -> Bus Creator1/9  "Vhcl Wheel RL rotv"
  Demux1/8 -> Bus Creator1/8  "Vhcl Wheel RL Trq_DL2WC"
  Demux1/7 -> Bus Creator1/7  "Vhcl Wheel RL Trq_B2WC"
  Demux1/6 -> Bus Creator1/6  "Vhcl Wheel FR rotv"
  Demux1/5 -> Bus Creator1/5  "Vhcl Wheel FR Trq_DL2WC"
  Demux1/4 -> Bus Creator1/4  "Vhcl Wheel FR Trq_B2WC"
  Demux1/3 -> Bus Creator1/3  "Vhcl Wheel FL rotv"
  In1/1 -> Demux1/1
  Bus Creator1/1 -> Out1/1
  Demux1/2 -> Bus Creator1/2  "Vhcl Wheel FL Trq_DL2WC"
  Demux1/1 -> Bus Creator1/1  "Vhcl Wheel FL Trq_B2WC"

== system SD2231_Lab1m/CarMaker/VehicleControl/CreateBus VhclCtrl ==
  In : Inport
  BusCreator : BusCreator  Inputs=29
  Demux : Demux  Outputs=29
  Out : Outport
  wires:
  In/1 -> Demux/1
  BusCreator/1 -> Out/1
  Demux/1 -> BusCreator/1  "VhclCtrl SST"
  Demux/2 -> BusCreator/2  "VhclCtrl Key"
  Demux/3 -> BusCreator/3  "VhclCtrl UserSignal0"
  Demux/4 -> BusCreator/4  "VhclCtrl UserSignal1"
  Demux/5 -> BusCreator/5  "VhclCtrl UserSignal2"
  Demux/6 -> BusCreator/6  "VhclCtrl UserSignal3"
  Demux/7 -> BusCreator/7  "VhclCtrl UserSignal4"
  Demux/8 -> BusCreator/8  "VhclCtrl GearNo"
  Demux/9 -> BusCreator/9  "VhclCtrl SelectorCtrl"
  Demux/10 -> BusCreator/10  "VhclCtrl Brake"
  Demux/11 -> BusCreator/11  "VhclCtrl BrakePark"
  Demux/12 -> BusCreator/12  "VhclCtrl Clutch"
  Demux/13 -> BusCreator/13  "VhclCtrl Gas"
  Demux/14 -> BusCreator/14  "VhclCtrl Steering Ang"
  Demux/15 -> BusCreator/15  "VhclCtrl Steering AngVel"
  Demux/16 -> BusCreator/16  "VhclCtrl Steering AngAcc"
  Demux/17 -> BusCreator/17  "VhclCtrl Steering Trq"
  Demux/18 -> BusCreator/18  "VhclCtrl Lights LowBeam"
  Demux/19 -> BusCreator/19  "VhclCtrl Lights HighBeam"
  Demux/20 -> BusCreator/20  "VhclCtrl Lights Daytime"
  Demux/21 -> BusCreator/21  "VhclCtrl Lights ParkL"
  Demux/22 -> BusCreator/22  "VhclCtrl Lights ParkR"
  Demux/23 -> BusCreator/23  "VhclCtrl Lights IndL"
  Demux/24 -> BusCreator/24  "VhclCtrl Lights IndR"
  Demux/25 -> BusCreator/25  "VhclCtrl Lights FogFrontL"
  Demux/26 -> BusCreator/26  "VhclCtrl Lights FogFrontR"
  Demux/27 -> BusCreator/27  "VhclCtrl Lights FogRear"
  Demux/28 -> BusCreator/28  "VhclCtrl Lights Brake"
  Demux/29 -> BusCreator/29  "VhclCtrl Lights Reverse"

== system SD2231_Lab1m/CarMaker/VehicleControl/CreateBus VhclCtrl.PT ==
  In1 : Inport
  BusCreator1 : BusCreator  Inputs=12
  Demux1 : Demux  Outputs=12
  Out1 : Outport
  wires:
  Demux1/12 -> BusCreator1/12  "VhclCtrl Brake"
  Demux1/11 -> BusCreator1/11  "VhclCtrl Gas"
  Demux1/10 -> BusCreator1/10  "VhclCtrl Clutch"
  Demux1/9 -> BusCreator1/9  "VhclCtrl SelectorCtrl"
  Demux1/8 -> BusCreator1/8  "VhclCtrl GearNo"
  Demux1/7 -> BusCreator1/7  "VhclCtrl UserSignal4"
  Demux1/6 -> BusCreator1/6  "VhclCtrl UserSignal3"
  Demux1/5 -> BusCreator1/5  "VhclCtrl UserSignal2"
  Demux1/4 -> BusCreator1/4  "VhclCtrl UserSignal1"
  Demux1/3 -> BusCreator1/3  "VhclCtrl UserSignal0"
  Demux1/2 -> BusCreator1/2  "VhclCtrl Key"
  Demux1/1 -> BusCreator1/1  "VhclCtrl SST"
  In1/1 -> Demux1/1
  BusCreator1/1 -> Out1/1

== system SD2231_Lab1m/CarMaker/VehicleControl/CreateBus VhclCtrl.Steering ==
  In1 : Inport
  Bus Creator : BusCreator  Inputs=5
  Demux : Demux  Outputs=5
  Out1 : Outport
  wires:
  In1/1 -> Demux/1
  Bus Creator/1 -> Out1/1
  Demux/1 -> Bus Creator/1  "VhclCtrl Steering Ang"
  Demux/5 -> Bus Creator/5  "VhclCtrl Steering SteerByTrq"
  Demux/3 -> Bus Creator/3  "VhclCtrl Steering AngAcc"
  Demux/2 -> Bus Creator/2  "VhclCtrl Steering AngVel"
  Demux/4 -> Bus Creator/4  "VhclCtrl Steering Trq"

== system SD2231_Lab1m/CarMaker/Your ABS Controller/ABS_PIDF ==
  In1 : Inport
  Derivative : Derivative
  Gain2 : Gain  Gain=Kp_brake
  Gain3 : Gain  Gain=Ki_brake
  Gain4 : Gain  Gain=Kd_brake
  Integrator : Integrator
  Sum2 : Sum  Inputs=|+++
  Out1 : Outport
  wires:
  Gain2/1 -> Sum2/3
  In1/1 -> Gain2/1, Gain4/1, Gain3/1
  Integrator/1 -> Sum2/2
  Derivative/1 -> Sum2/1
  Gain4/1 -> Derivative/1
  Gain3/1 -> Integrator/1
  Sum2/1 -> Out1/1

== system SD2231_Lab1m/CarMaker/Your ABS Controller/ABS_PIDR ==
  In1 : Inport
  Derivative : Derivative
  Gain2 : Gain  Gain=Kp_brake_r
  Gain3 : Gain  Gain=Ki_brake_r
  Gain4 : Gain  Gain=Kd_brake_r
  Integrator : Integrator
  Sum2 : Sum  Inputs=|+++
  Out1 : Outport
  wires:
  Gain2/1 -> Sum2/3
  In1/1 -> Gain4/1, Gain3/1, Gain2/1
  Integrator/1 -> Sum2/2
  Derivative/1 -> Sum2/1
  Gain4/1 -> Derivative/1
  Gain3/1 -> Integrator/1
  Sum2/1 -> Out1/1

== system SD2231_Lab1m/CarMaker/Your Traction Controller/TCS_PID ==
  In1 : Inport
  Derivative : Derivative
  Gain2 : Gain  Gain=Kp_em
  Gain3 : Gain  Gain=Ki_em
  Gain4 : Gain  Gain=Kd_em
  Integrator : Integrator
  Sum2 : Sum  Inputs=|+++
  Out1 : Outport
  wires:
  Gain2/1 -> Sum2/3
  In1/1 -> Gain4/1, Gain3/1, Gain2/1
  Integrator/1 -> Sum2/2
  Derivative/1 -> Sum2/1
  Gain4/1 -> Derivative/1
  Gain3/1 -> Integrator/1
  Sum2/1 -> Out1/1

== system SD2231_Lab1m/CarMaker/Your observer/FL_observer ==
  <Vehicle velocity> : Inport
  <FL Tyre rot vel> : Inport  Port=2
  <FL Tyre radius> : Inport  Port=3
  Braking Slip : Product  Inputs=***/
  Constant : Constant  Value=0
  Constant1 : Constant  Value=-1
  Fcn : Fcn  Expr=u+(u==0)*eps
  Fcn1 : Fcn  Expr=u+(u==0)*eps
  Linear : simulink/Logic and Bit Operations/Compare To Constant  relop=>=  const=1  OutDataTypeStr=boolean
  Multiply : Product
  Multiply1 : Product
  NOT : Logic  Operator=NOT  IconShape=distinctive  AllPortsSameDT=off
  Relational Operator : RelationalOperator  RndMeth=Simplest
  "Rotational " : simulink/Logic and Bit Operations/Compare To Constant  relop=>=  const=3  OutDataTypeStr=boolean
  Sum : Sum  Inputs=|-+
  Traction Slip : Product  Inputs=***/
  FL_BS : Outport
  FL_TS : Outport  Port=2
  wires:
  Braking Slip/1 -> FL_BS/1
  <FL Tyre radius>/1 -> Multiply/2
  <FL Tyre rot vel>/1 -> Multiply/1, "Rotational "/1
  Sum/1 -> Traction Slip/3, Relational Operator/1, Multiply1/1
  Constant/1 -> Relational Operator/2
  Constant1/1 -> Multiply1/2
  NOT/1 -> Braking Slip/1
  Linear/1 -> Braking Slip/2
  "Rotational "/1 -> Traction Slip/2
  Multiply1/1 -> Braking Slip/3
  <Vehicle velocity>/1 -> Linear/1, Fcn/1, Sum/1
  Multiply/1 -> Fcn1/1, Sum/2
  Traction Slip/1 -> FL_TS/1
  Relational Operator/1 -> Traction Slip/1, NOT/1
  Fcn1/1 -> Traction Slip/4
  Fcn/1 -> Braking Slip/4

== system SD2231_Lab1m/CarMaker/Your observer/FR_observer ==
  <Vehicle velocity> : Inport
  <FR_RL Tyre rot vel> : Inport  Port=2
  <FR_RL Tyre radius> : Inport  Port=3
  Braking Slip : Product  Inputs=***/
  Constant : Constant  Value=0
  Constant1 : Constant  Value=-1
  Fcn : Fcn  Expr=u+(u==0)*eps
  Fcn1 : Fcn  Expr=u+(u==0)*eps
  Linear : simulink/Logic and Bit Operations/Compare To Constant  relop=>=  const=0.9  OutDataTypeStr=boolean
  Multiply : Product
  Multiply1 : Product
  NOT : Logic  Operator=NOT  IconShape=distinctive  AllPortsSameDT=off
  Relational Operator : RelationalOperator  RndMeth=Simplest
  "Rotational " : simulink/Logic and Bit Operations/Compare To Constant  relop=>=  const=3  OutDataTypeStr=boolean
  Sum : Sum  Inputs=|-+
  Traction Slip : Product  Inputs=***/
  FR_BS : Outport
  FR_TS : Outport  Port=2
  wires:
  Braking Slip/1 -> FR_BS/1
  <FR_RL Tyre radius>/1 -> Multiply/2
  <FR_RL Tyre rot vel>/1 -> Multiply/1, "Rotational "/1
  Sum/1 -> Traction Slip/3, Relational Operator/1, Multiply1/1
  Constant/1 -> Relational Operator/2
  Constant1/1 -> Multiply1/2
  NOT/1 -> Braking Slip/1
  Linear/1 -> Braking Slip/2
  "Rotational "/1 -> Traction Slip/2
  Multiply1/1 -> Braking Slip/3
  <Vehicle velocity>/1 -> Linear/1, Fcn/1, Sum/1
  Multiply/1 -> Fcn1/1, Sum/2
  Traction Slip/1 -> FR_TS/1
  Relational Operator/1 -> Traction Slip/1, NOT/1
  Fcn/1 -> Braking Slip/4
  Fcn1/1 -> Traction Slip/4

== system SD2231_Lab1m/CarMaker/Your observer/RL_observer ==
  <Vehicle velocity> : Inport
  <RL Tyre rot vel> : Inport  Port=2
  <RL Tyre radius> : Inport  Port=3
  Braking Slip : Product  Inputs=***/
  Constant : Constant  Value=0
  Constant1 : Constant  Value=-1
  Fcn : Fcn  Expr=u+(u==0)*eps
  Fcn1 : Fcn  Expr=u+(u==0)*eps
  Linear : simulink/Logic and Bit Operations/Compare To Constant  relop=>=  const=0.9  OutDataTypeStr=boolean
  Multiply : Product
  Multiply1 : Product
  NOT : Logic  Operator=NOT  IconShape=distinctive  AllPortsSameDT=off
  Relational Operator : RelationalOperator  RndMeth=Simplest
  "Rotational " : simulink/Logic and Bit Operations/Compare To Constant  relop=>=  const=1  OutDataTypeStr=boolean
  Sum : Sum  Inputs=|-+
  Traction Slip : Product  Inputs=***/
  RL_BS : Outport
  RL_TS : Outport  Port=2
  wires:
  Braking Slip/1 -> RL_BS/1
  <RL Tyre radius>/1 -> Multiply/2
  <RL Tyre rot vel>/1 -> Multiply/1, "Rotational "/1
  Sum/1 -> Traction Slip/3, Relational Operator/1, Multiply1/1
  Constant/1 -> Relational Operator/2
  Constant1/1 -> Multiply1/2
  NOT/1 -> Braking Slip/1
  Linear/1 -> Braking Slip/2
  "Rotational "/1 -> Traction Slip/2
  Multiply1/1 -> Braking Slip/3
  <Vehicle velocity>/1 -> Linear/1, Fcn/1, Sum/1
  Multiply/1 -> Fcn1/1, Sum/2
  Traction Slip/1 -> RL_TS/1
  Relational Operator/1 -> Traction Slip/1, NOT/1
  Fcn1/1 -> Traction Slip/4
  Fcn/1 -> Braking Slip/4

== system SD2231_Lab1m/CarMaker/Your observer/RR_observer ==
  <Vehicle velocity> : Inport
  <RR Tyre rot vel> : Inport  Port=2
  <RR Tyre radius> : Inport  Port=3
  Braking Slip : Product  Inputs=***/
  Constant : Constant  Value=0
  Constant1 : Constant  Value=-1
  Fcn : Fcn  Expr=u+(u==0)*eps
  Fcn1 : Fcn  Expr=u+(u==0)*eps
  Linear : simulink/Logic and Bit Operations/Compare To Constant  relop=>=  const=0.9  OutDataTypeStr=boolean
  Multiply : Product
  Multiply1 : Product
  NOT : Logic  Operator=NOT  IconShape=distinctive  AllPortsSameDT=off
  Relational Operator : RelationalOperator  RndMeth=Simplest
  "Rotational " : simulink/Logic and Bit Operations/Compare To Constant  relop=>=  const=3  OutDataTypeStr=boolean
  Sum : Sum  Inputs=|-+
  Traction Slip : Product  Inputs=***/
  RR_BS : Outport
  RR_TS : Outport  Port=2
  wires:
  Braking Slip/1 -> RR_BS/1
  <RR Tyre radius>/1 -> Multiply/2
  <RR Tyre rot vel>/1 -> Multiply/1, "Rotational "/1
  Sum/1 -> Traction Slip/3, Relational Operator/1, Multiply1/1
  Constant/1 -> Relational Operator/2
  Constant1/1 -> Multiply1/2
  NOT/1 -> Braking Slip/1
  Linear/1 -> Braking Slip/2
  "Rotational "/1 -> Traction Slip/2
  Multiply1/1 -> Braking Slip/3
  <Vehicle velocity>/1 -> Linear/1, Fcn/1, Sum/1
  Multiply/1 -> Fcn1/1, Sum/2
  Traction Slip/1 -> RR_TS/1
  Relational Operator/1 -> Traction Slip/1, NOT/1
  Fcn/1 -> Braking Slip/4
  Fcn1/1 -> Traction Slip/4

== system SD2231_Lab1m/CarMaker/IPG Vehicle/Brake1/CreateBus Vhcl.Wheel.PT ==
  In : Inport
  BusCreator1 : BusCreator  Inputs=20
  Demux1 : Demux  Outputs=20
  Out : Outport
  wires:
  Demux1/20 -> BusCreator1/20  "Vhcl Trq_DriveSrc_trg d3"
  Demux1/19 -> BusCreator1/19  "Vhcl Trq_DriveSrc_trg d2"
  Demux1/18 -> BusCreator1/18  "Vhcl Trq_DriveSrc_trg d1"
  Demux1/17 -> BusCreator1/17  "Vhcl Trq_DriveSrc_trg d0"
  Demux1/16 -> BusCreator1/16  "Vhcl Wheel RR WhlBearing"
  Demux1/15 -> BusCreator1/15  "Vhcl Wheel RR Trq_T2W"
  Demux1/14 -> BusCreator1/14  "Vhcl Wheel RR Trq_BrakeReg_trg"
  Demux1/13 -> BusCreator1/13  "Vhcl Wheel RR Trq_Brake"
  Demux1/12 -> BusCreator1/12  "Vhcl Wheel RL WhlBearing"
  Demux1/11 -> BusCreator1/11  "Vhcl Wheel RL Trq_T2W"
  Demux1/10 -> BusCreator1/10  "Vhcl Wheel RL Trq_BrakeReg_trg"
  Demux1/9 -> BusCreator1/9  "Vhcl Wheel RL Trq_Brake"
  Demux1/8 -> BusCreator1/8  "Vhcl Wheel FR WhlBearing"
  Demux1/7 -> BusCreator1/7  "Vhcl Wheel FR Trq_T2W"
  Demux1/6 -> BusCreator1/6  "Vhcl Wheel FR Trq_BrakeReg_trg"
  Demux1/5 -> BusCreator1/5  "Vhcl Wheel FR Trq_Brake"
  Demux1/4 -> BusCreator1/4  "Vhcl Wheel FL WhlBearing"
  Demux1/3 -> BusCreator1/3  "Vhcl Wheel FL Trq_T2W"
  Demux1/2 -> BusCreator1/2  "Vhcl Wheel FL Trq_BrakeReg_trg"
  Demux1/1 -> BusCreator1/1  "Vhcl Wheel FL Trq_Brake"
  BusCreator1/1 -> Out/1
  In/1 -> Demux1/1

== system SD2231_Lab1m/CarMaker/IPG Vehicle/Brake1/UserDefinedBrakingSystem ==
  note: Please note: Influence of DrivMan.Handbrake on the braking
      | torques (Brake IF Trq_XX signals) is ignored in this example.
  SD2231.Data : Inport
  Bus Creator2 : BusCreator  Inputs=16
  Bus Selector : BusSelector  OutputSignals=FLBrakeAdjust,FRBrakeAdjust,RLBrakeAdjust,RRBrakeAdjust
  Constant : Constant  Value=0
  NOTSET : Constant  Value=-99999
  Subsystem : Subsystem
  Subsystem1 : Subsystem
  Subsystem2 : Subsystem
  Subsystem3 : Subsystem
  Brake.IF.Out : Outport
  wires:
  SD2231.Data/1 -> Bus Selector/1
  Bus Creator2/1 -> Brake.IF.Out/1
  Constant/1 -> Bus Creator2/10, Bus Creator2/5, Bus Creator2/6, Bus Creator2/7, Bus Creator2/8, Bus Creator2/9, Bus Creator2/11, Bus Creator2/12
  NOTSET/1 -> Bus Creator2/13, Bus Creator2/14, Bus Creator2/15, Bus Creator2/16
  Subsystem/1(FL brake force) -> Bus Creator2/1
  Bus Selector/1 -> Subsystem/1(FLBrakeAdjust)  "<FLBrakeAdjust>"
  Subsystem1/1(FR brake force) -> Bus Creator2/2
  Subsystem2/1(RL brake force) -> Bus Creator2/3
  Subsystem3/1(RR brake force) -> Bus Creator2/4
  Bus Selector/2 -> Subsystem1/1(FRBrakeAdjust)  "<FRBrakeAdjust>"
  Bus Selector/3 -> Subsystem2/1(RLBrakeAdjust)  "<RLBrakeAdjust>"
  Bus Selector/4 -> Subsystem3/1(RRBrakeAdjust)  "<RRBrakeAdjust>"

== system SD2231_Lab1m/CarMaker/IPG Vehicle/CarAndTrailer1/CarAndTrailerUpd ==
  Sync_In : Inport
  Vhcl.Steering : Inport  Port=2
  Vhcl.Motion : Inport  Port=3
  Vhcl.PoI : Inport  Port=4
  Vhcl.Wheel.FL : Inport  Port=5
  Vhcl.Wheel.FR : Inport  Port=6
  Vhcl.Wheel.RL : Inport  Port=7
  Vhcl.Wheel.RR : Inport  Port=8
  Car.Hitch.FrcTrq : Inport  Port=9
  Vhcl.Fr1A : Inport  Port=10
  CarAndTrailerUpd : S-Function  FunctionName=CM_Sfun  Parameters='CarAndTrUpd'  SFunctionDeploymentMode=off  EnableBusSupport=off
  CreateBus Brake.IF.In : Subsystem
  Sync_Out : Outport
  Brake.IF.In : Outport  Port=2
  wires:
  Vhcl.Fr1A/1 -> CarAndTrailerUpd/10  "user vehicle only"
  Vhcl.Steering/1 -> CarAndTrailerUpd/2
  Vhcl.Motion/1 -> CarAndTrailerUpd/3
  Vhcl.PoI/1 -> CarAndTrailerUpd/4
  Vhcl.Wheel.FL/1 -> CarAndTrailerUpd/5
  Vhcl.Wheel.FR/1 -> CarAndTrailerUpd/6
  Car.Hitch.FrcTrq/1 -> CarAndTrailerUpd/9
  Vhcl.Wheel.RR/1 -> CarAndTrailerUpd/8
  Vhcl.Wheel.RL/1 -> CarAndTrailerUpd/7
  CarAndTrailerUpd/2 -> CreateBus Brake.IF.In/1(In)
  CreateBus Brake.IF.In/1(Out) -> Brake.IF.In/1
  CarAndTrailerUpd/1 -> Sync_Out/1
  Sync_In/1 -> CarAndTrailerUpd/1

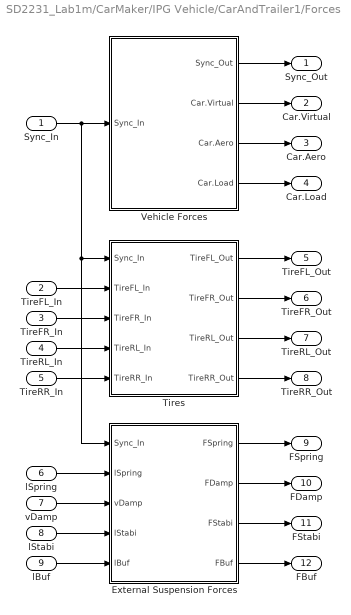
== system SD2231_Lab1m/CarMaker/IPG Vehicle/CarAndTrailer1/Forces ==
  Sync_In : Inport
  TireFL_In : Inport  Port=2
  TireFR_In : Inport  Port=3
  TireRL_In : Inport  Port=4
  TireRR_In : Inport  Port=5
  lSpring : Inport  Port=6
  vDamp : Inport  Port=7
  lStabi : Inport  Port=8
  lBuf : Inport  Port=9
  External Suspension Forces : Subsystem
  Tires : Subsystem
  Vehicle Forces : Subsystem
  Sync_Out : Outport
  Car.Virtual : Outport  Port=2
  Car.Aero : Outport  Port=3
  Car.Load : Outport  Port=4
  TireFL_Out : Outport  Port=5
  TireFR_Out : Outport  Port=6
  TireRL_Out : Outport  Port=7
  TireRR_Out : Outport  Port=8
  FSpring : Outport  Port=9
  FDamp : Outport  Port=10
  FStabi : Outport  Port=11
  FBuf : Outport  Port=12
  wires:
  lBuf/1 -> External Suspension Forces/5(lBuf)
  lStabi/1 -> External Suspension Forces/4(lStabi)
  vDamp/1 -> External Suspension Forces/3(vDamp)
  Tires/4(TireRR_Out) -> TireRR_Out/1
  Tires/3(TireRL_Out) -> TireRL_Out/1
  Tires/2(TireFR_Out) -> TireFR_Out/1
  Tires/1(TireFL_Out) -> TireFL_Out/1
  TireRR_In/1 -> Tires/5(TireRR_In)
  TireRL_In/1 -> Tires/4(TireRL_In)
  TireFR_In/1 -> Tires/3(TireFR_In)
  TireFL_In/1 -> Tires/2(TireFL_In)
  External Suspension Forces/4(FBuf) -> FBuf/1
  Sync_In/1 -> External Suspension Forces/1(Sync_In), Tires/1(Sync_In), Vehicle Forces/1(Sync_In)
  Vehicle Forces/1(Sync_Out) -> Sync_Out/1
  Vehicle Forces/2(Car.Virtual) -> Car.Virtual/1
  Vehicle Forces/3(Car.Aero) -> Car.Aero/1
  Vehicle Forces/4(Car.Load) -> Car.Load/1
  lSpring/1 -> External Suspension Forces/2(lSpring)
  External Suspension Forces/2(FDamp) -> FDamp/1
  External Suspension Forces/3(FStabi) -> FStabi/1
  External Suspension Forces/1(FSpring) -> FSpring/1

== system SD2231_Lab1m/CarMaker/IPG Vehicle/CarAndTrailer1/Kinematics ==
  Sync_In : Inport
  Steer.IF : Inport  Port=2
  Kinematics : S-Function  FunctionName=CM_Sfun  Parameters='Kinematics'  SFunctionDeploymentMode=off  EnableBusSupport=off
  Sync_Out : Outport
  TireFL_In : Outport  Port=2
  TireFR_In : Outport  Port=3
  TireRL_In : Outport  Port=4
  TireRR_In : Outport  Port=5
  lSpring : Outport  Port=6
  vDamp : Outport  Port=7
  lStabi : Outport  Port=8
  lBuf : Outport  Port=9
  wires:
  Kinematics/9 -> lBuf/1
  Kinematics/8 -> lStabi/1
  Kinematics/2 -> TireFL_In/1
  Kinematics/3 -> TireFR_In/1
  Kinematics/4 -> TireRL_In/1
  Kinematics/5 -> TireRR_In/1
  Kinematics/6 -> lSpring/1
  Kinematics/7 -> vDamp/1
  Sync_In/1 -> Kinematics/1
  Kinematics/1 -> Sync_Out/1
  Steer.IF/1 -> Kinematics/2
